simulink model "MultiportSwitch_TestGen6"  (R2017b)
settings: Solver=FixedStepDiscrete  StartTime=0.0  StopTime=10.0  RelTol=1e-3
settings Model: Creator=ktrinh  LastModifiedBy=ktrinh
settings DebuggingCC: ParameterOverflowMsg=none

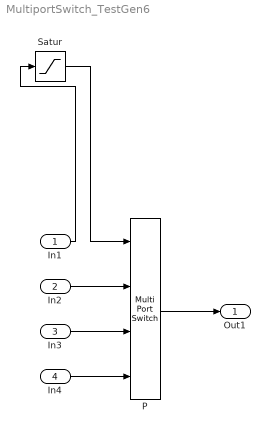
== system MultiportSwitch_TestGen6 ==
  In1 : Inport  OutMin=0  OutMax=2
  In2 : Inport  Port=2  PortDimensions=[2,3]
  In3 : Inport  Port=3  PortDimensions=[2,3]
  In4 : Inport  Port=4  PortDimensions=[2,3]
  P : MultiPortSwitch  DataPortOrder=Zero-based contiguous  Inputs=2  DataPortForDefault=Additional data port
  Satur : Saturate  UpperLimit=2  LowerLimit=0
  Out1 : Outport
  wires:
  In2/1 -> P/2
  In3/1 -> P/3
  In4/1 -> P/4
  P/1 -> Out1/1
  In1/1 -> Satur/1
  Satur/1 -> P/1
